simulink library "Lib_Turbo_Ambient_TMATS_org"  (Simulink 10.0)
settings: Solver=ode45  StartTime=0.0  StopTime=10.0  RelTol=1e-3  EnableMultiTasking=on
Description:
  | Thomas Modules
settings Model: Creator=jwchapm2  LastModifiedBy=bhisma

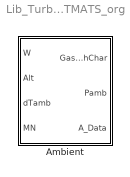
== system Lib_Turbo_Ambient_TMATS_org ==
  Ambient : Subsystem  mask(T-MATS: Ambient Library Block){X_A_AltVec_M=5000*[-1 0 1 2 3 4 5 6 7 8 9 10 12 14 16], T_A_TsVec_M=[536.51 518.67 500.84 483.03 465.22 447.41 429.62 411.84 394.06 389.97 389.97 389.97 389.97 392.25 397.69], T_A_PsVec_M=[17.554 14.696 12.228 10.108 8.297 6.759 5.461 4.373 3.468 2.73 2.149 1.692 1.049 0.651 0.406], AFARc_M=0, X_A_FARVec_M=[0; 0.0050; 0.0100; 0.0150; 0.0200; 0.0250; 0.0300], T_A_RtArray_M=[0.0686;    0.0686;    0.0686;    0.0686;    0.0686;    0.0686;    0.0686], Y_A_TVec_M=[300 10000], T_A_gammaArray_M=[ 1.4 1.4 1.4 1.4 1.4 1.4 1.4; 1.4 1.4 1.4 1.4 1.4 1.4 1.4]}
      mask prompts: X_A_AltVec_M "X_A_AltVec_M - Ambient Altitude Vector (mx1)"; T_A_TsVec_M "T_A_TsVec_M - Ambient Static Temperature Table Vector (Ts = f(Alt)) (mx1)"; T_A_PsVec_M "T_A_PsVec_M - Ambient Static Pressure Table Vector (Ps = f(Alt)) (mx1)"; AFARc_M "AFARc_M - Ambient air quality (combusted Fuel to Air Ratio) [frac]"; X_A_FARVec_M "X_A_FARVec_M - Fuel to Air ratio Vector (fx1)"; T_A_RtArray_M "T_A_RtArray_M - Rt Table (Rt = f(FAR)) (fx1)"; Y_A_TVec_M "Y_A_TVec_M - Temperature  Vector (tx1)"; T_A_gammaArray_M "T_A_gammaArray_M - gamma Table (gamma = f(T,FAR)) (txf)"
      mask help: This block translates environmental condition to gas characteristics: Alt, dTamb, Air purity, and MN to Pressure, Temperature, FAR, and Velocity.
      mask Help: web(which('Turbo_TMATS_Amb.html'),'-helpbrowser')

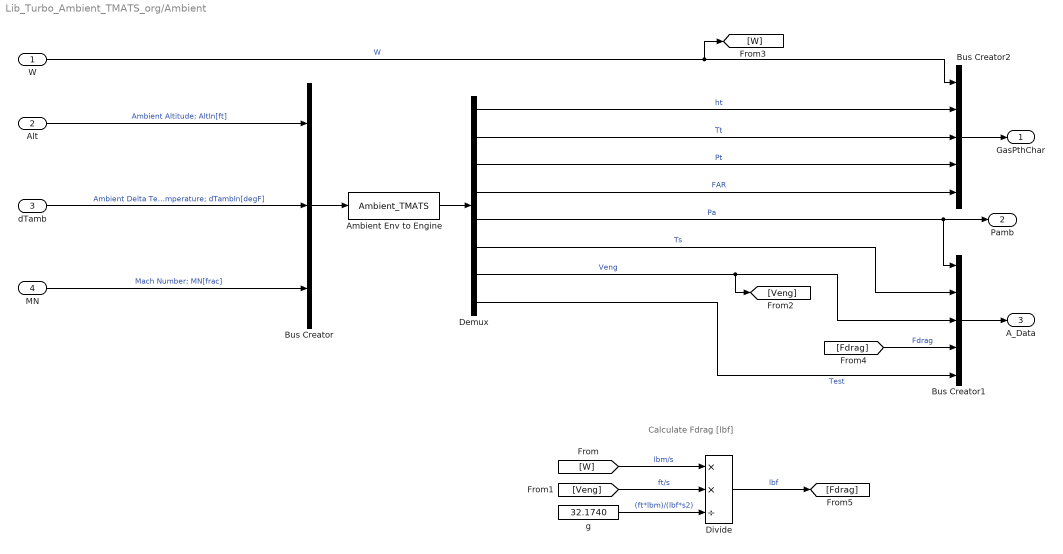
== system Lib_Turbo_Ambient_TMATS_org/Ambient ==
  note: Calculate Fdrag [lbf]
  W : Inport
  Alt : Inport  Port=2
  dTamb : Inport  Port=3
  MN : Inport  Port=4
  Ambient Env to Engine : S-Function  FunctionName=Ambient_TMATS  Parameters="X_A_AltVec_M, T_A_TsVec_M, T_A_PsVec_M, X_A_FARVec_M, Y_A_TVec_M, T_A_RtArray_M, T_A_gammaArray_M, AFARc_M,   gcs"  SFunctionModules='pt2sc_TMATS sp2tc_TMATS t2hc_TMATS interp1Ac_TMATS interp2Ac_TMATS functions_TMATS'  SFunctionDeploymentMode=off  EnableBusSupport=off
  Bus Creator : BusCreator  Inputs=3
  Bus Creator1 : BusCreator  Inputs=5
  Bus Creator2 : BusCreator  Inputs=5
  Demux : Demux  Outputs=8
  Divide : Product  Inputs=**/
  g : Constant  Value=32.1740
  GasPthChar : Outport
  Pamb : Outport  Port=2
  A_Data : Outport  Port=3
  wires:
  Demux/6 -> Bus Creator1/2  "Ts"
  Demux/5 -> Bus Creator1/1, Pamb/1  "Pa"
  Ambient Env to Engine/1 -> Demux/1
  Demux/2 -> Bus Creator2/3  "Tt"
  Demux/3 -> Bus Creator2/4  "Pt"
  Bus Creator/1 -> Ambient Env to Engine/1
  dTamb/1 -> Bus Creator/2  "Ambient Delta Temperature; dTambIn[degF]"
  MN/1 -> Bus Creator/3  "Mach Number; MN[frac]"
  Alt/1 -> Bus Creator/1  "Ambient Altitude; AltIn[ft]"
  Demux/7 -> [Veng], Bus Creator1/3  "Veng"
  Demux/4 -> Bus Creator2/5  "FAR"
  Bus Creator1/1 -> A_Data/1
  Demux/1 -> Bus Creator2/2  "ht"
  W/1 -> [W], Bus Creator2/1  "W"
  Bus Creator2/1 -> GasPthChar/1
  Demux/8 -> Bus Creator1/5  "Test"
  g/1 -> Divide/3  "(ft*lbm)/(lbf*s2)"
  [Veng] -> Divide/2  "ft/s"
  [W] -> Divide/1  "lbm/s"
  Divide/1 -> [Fdrag]  "lbf"
  [Fdrag] -> Bus Creator1/4  "Fdrag"
